simulink model "ModelB"  (R2018a)
settings: Solver=ode23  StartTime=0.0  StopTime=0.25  MaxStep=10e-6  RelTol=1e-3
libraries: powerlib x13, powerlib_meascontrol x1
settings Model: Creator=ivank  LastModifiedBy=ivank
settings SolverCC: InitialStep=10e-8

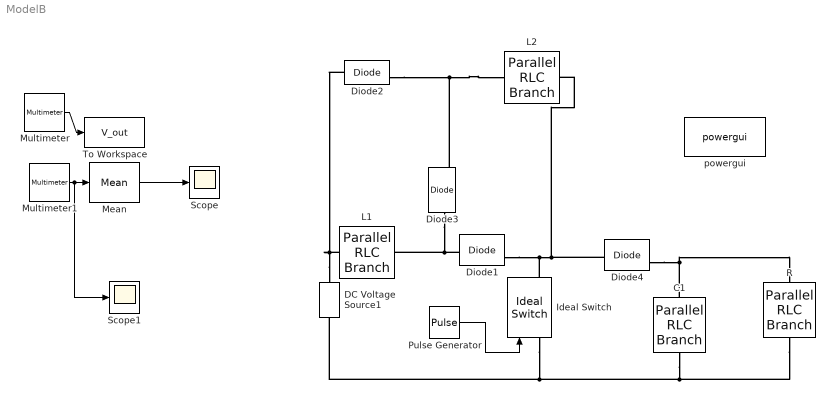
== system ModelB ==
  "C1 " : powerlib/Elements/Parallel RLC Branch  LConnTagsString=a  RConnTagsString=__new0  BranchType=C  Resistance=7.225  Inductance=150e-6  SetiL0=off  InitialCurrent=0  Capacitance=220e-6  Setx0=off  InitialVoltage=0  Measurements=Branch voltage and current
  DC Voltage Source1 : powerlib/Electrical Sources/DC Voltage Source  Amplitude=10  Measurements=None
  Diode{1..4} (4 alike) : powerlib/Power Electronics/Diode  Ron=0.001  Lon=0  Vf=0  IC=0  UseSnubber=0  Rs=500  Cs=250e-9  Measurements=on
  Ideal Switch : powerlib/Power Electronics/Ideal Switch  Ron=0.001  Lon=0  IC=0  Rs=1e5  Cs=inf  Measurements=on
  L1 : powerlib/Elements/Parallel RLC Branch  LConnTagsString=a  RConnTagsString=__new0  BranchType=L  Resistance=7.225  Inductance=150e-6  SetiL0=off  InitialCurrent=0  Capacitance=100*10e-6  Setx0=off  InitialVoltage=0  Measurements=Branch voltage and current
  L2 : powerlib/Elements/Parallel RLC Branch  LConnTagsString=a  RConnTagsString=__new0  BranchType=L  Resistance=7.225  Inductance=700e-6  SetiL0=off  InitialCurrent=0  Capacitance=100*10e-6  Setx0=off  InitialVoltage=0  Measurements=Branch voltage and current
  Mean : powerlib_meascontrol/Measurements/Mean  Freq=60  Vinit=0  Ts=0
  Multimeter : powerlib/Measurements/Multimeter  PhasorSimulation=off  OutputType=Complex  sel=4  L=8  Gain=1  yselected={'Ub: R '};  PSBOutputType=1  PSBequivalent=0  AxesSetting=[0,0.1,-100,100]  Display=1  SavedBlockNames=-11
  Multimeter1 : powerlib/Measurements/Multimeter  PhasorSimulation=off  OutputType=Complex  sel=4  L=8  Gain=1  yselected={'Ub: R '};  PSBOutputType=1  PSBequivalent=0  AxesSetting=[0,0.1,-100,100]  Display=0  SavedBlockNames=-11
  Pulse Generator : DiscretePulseGenerator  PulseType=Time based  Period=1/50000  PulseWidth=50
  "R " : powerlib/Elements/Parallel RLC Branch  LConnTagsString=a  RConnTagsString=__new0  BranchType=R  Resistance=225  Inductance=1e-3  SetiL0=off  InitialCurrent=0  Capacitance=100*10e-6  Setx0=off  InitialVoltage=0  Measurements=Branch voltage and current
  Scope : Scope
  Scope1 : Scope
  To Workspace : ToWorkspace  VariableName=V_out  SaveFormat=Timeseries  SampleTime=-1
  powergui : powerlib/powergui  Priority=1  SimulationMode=Continuous  SampleTime=50e-6  frequency=60  Iterations=50  frequencyindice=0  Pbase=100e6  ErrMax=1e-4  UnitsV=kV  UnitsW=MW  buscounter=0  FunctionMessages=off  echomessages=off  EnableUseOfTLC=off  CurrentSourceSwitches=off  DisableSnubberDevices=off  DisableRonSwitches=off  DisableVfSwitches=off  DisplayEquations=off  SolverType=Tustin/Backward Euler (TBE)  Interpol=off  ExternalGateDelay=off  methode=off  Ts=100  x0status=blocks  SPID=on  SwTol=0  HookPort=off  RestoreLinks=warning  ResistiveCurrentMeasurement=off  Frange=[0:2:500]  Ylog=off  Xlog=on  ShowGrid=off  save=off  variable=ZData  structure=0  ZoomFFT=off  StartTime=0.0  cycles=1  DisplayStyle=1  fundamental=60  FreqAxis=off  MaxFrequency=1000  frequencyindicesteady=1  RmsSteady=1  display=off
  wires:
  Pulse Generator/1 -> Ideal Switch/1
  Multimeter1/1 -> Scope1/1, Mean/1
  Mean/1 -> Scope/1
  Multimeter/1 -> To Workspace/1
  connections:
  DC Voltage Source1/LConn1 -- "R "/RConn1 -- "C1 "/RConn1 -- Ideal Switch/LConn1
  DC Voltage Source1/RConn1 -- L1/RConn1 -- Diode2/LConn1
  Diode3/LConn1 -- L1/LConn1 -- Diode1/LConn1
  Diode2/RConn1 -- Diode3/RConn1 -- L2/RConn1
  Diode1/RConn1 -- Ideal Switch/RConn1 -- Diode4/LConn1 -- L2/LConn1
  "C1 "/LConn1 -- Diode4/RConn1 -- "R "/LConn1
